simulink model "model_plane_identification_script_v1"  (R2015b)
settings: Solver=FixedStepDiscrete  StartTime=0.0  StopTime=20  RelTol=1e-3
values from neighbouring files (symbols this model uses):
  Aa = Amp_list(ii)    [amplitude_influence.m]    (also in datas.m = 1; model_validation.m = Amp_aileron2)
  Ae = Amp_list(ii)    [amplitude_influence.m]    (also in datas.m = 1; model_validation.m = Amp_elevator2)
  Ar = Amp_list(ii)    [amplitude_influence.m]    (also in datas.m = 1; model_validation.m = Amp_rudder2)
  b = 59.74    [datas.m]
  cbar = 8.32    [datas.m]
  K_wind = [0 0 0 0 0 0]'    [datas.m]
  m = 288772    [datas.m]
  Offset_Accelerometer = 57*10^-6    (= 5.7e-05)    [datas.m]
  Offset_gyro = 0.15/180*pi    (= 0.00261799387799)    [datas.m]
  Offset_velocity_angles = 0.1/180*pi    (= 0.00174532925199)    [datas.m]
  S = 510.95    [datas.m]
  Ta = 6    [datas.m]
  Te = 4    [datas.m]
  test_aileron = 1    [datas.m]    (also in model_validation.m = aileron2)
  test_elevator = 4    [datas.m]    (also in model_validation.m = elevator2)
  test_rudder = 1    [datas.m]    (also in model_validation.m = rudder2)
  Tr = 2    [datas.m]
undefined symbols (not defined in the file or in its folder): airlib, B747, DiscIntNeverNeededParam, DT, sigbuilder_block
undefined symbols (not defined in the file): Cd_0_true, Cd_alpha_true, Cd_deltae_true, Cd_q_true, Cdih_true, Cl_0_true, CL_0_true, CL_alpha_true, Cl_b_true, Cl_deltaa_true, CL_deltae_true, Cl_deltar_true, Cl_p_true, CL_q_true, Cl_r_true, CLih_true, Cm_0_true, Cm_alpha_true, Cm_deltae_true, Cm_ih_true, Cm_q_true, Cn_0_true, Cn_b_true, Cn_deltaa_true, Cn_deltar_true, Cn_p_true, Cn_r_true, Cy_0_true, Cy_b_true, Cy_deltaa_true, Cy_deltar_true, Cy_p_true, Cy_r_true, Ix, Iy, Iz, Jxy, Jxz, Jyz, V
libraries: simulink x4
(part 2 of 2)

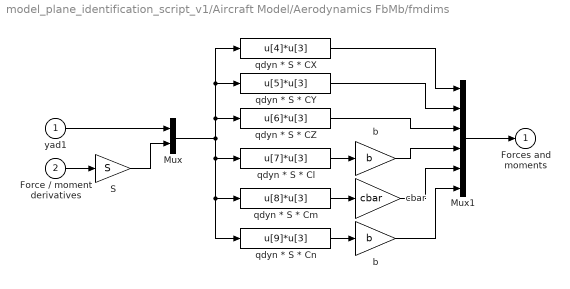
== system model_plane_identification_script_v1/Aircraft Model/Aerodynamics FbMb/fmdims ==
  yad1 : Inport
  Force / moment derivatives : Inport  Port=2
  Mux : Mux  Inputs=[3 6]
  Mux1 : Mux  Inputs=6
  S : Gain  Gain=S  SaturateOnIntegerOverflow=on  OutDataTypeStr=Inherit: Same as input  ParamDataTypeStr=Inherit: Same as input
  b : Gain  Gain=b  SaturateOnIntegerOverflow=on  OutDataTypeStr=Inherit: Same as input  ParamDataTypeStr=Inherit: Same as input
  "b " : Gain  Gain=b  SaturateOnIntegerOverflow=on  OutDataTypeStr=Inherit: Same as input  ParamDataTypeStr=Inherit: Same as input
  cbar : Gain  Gain=cbar  SaturateOnIntegerOverflow=on  OutDataTypeStr=Inherit: Same as input  ParamDataTypeStr=Inherit: Same as input
  qdyn * S * CX : Fcn  Expr=u[4]*u[3]
  qdyn * S * CY : Fcn  Expr=u[5]*u[3]
  qdyn * S * CZ : Fcn  Expr=u[6]*u[3]
  qdyn * S * Cl : Fcn  Expr=u[7]*u[3]
  qdyn * S * Cm : Fcn  Expr=u[8]*u[3]
  qdyn * S * Cn : Fcn  Expr=u[9]*u[3]
  Forces and moments : Outport
  wires:
  b/1 -> Mux1/4
  qdyn * S * CZ/1 -> Mux1/3
  S/1 -> Mux/2
  qdyn * S * CY/1 -> Mux1/2
  qdyn * S * CX/1 -> Mux1/1
  yad1/1 -> Mux/1
  qdyn * S * Cn/1 -> "b "/1
  qdyn * S * Cm/1 -> cbar/1
  qdyn * S * Cl/1 -> b/1
  Mux/1 -> qdyn * S * Cn/1, qdyn * S * Cm/1, qdyn * S * Cl/1, qdyn * S * CY/1, qdyn * S * CX/1, qdyn * S * CZ/1
  Force / moment derivatives/1 -> S/1
  cbar/1 -> Mux1/5
  "b "/1 -> Mux1/6
  Mux1/1 -> Forces and moments/1

== system model_plane_identification_script_v1/Aircraft Model/Aircraft equations of motion (General)/ODE ==
  x : Inport
  Ftot : Inport  Port=2
  Mtot : Inport  Port=3
  yhlp : Inport  Port=4
  ybvel* : Inport  Port=5
  Eulerdot : Subsystem  mask(Eulerdot){}
      mask help:
      | Calculation of d(psi)/dt, d(theta)/dt,
      | and d(phi/dt)
      mask Display: disp('psi dot\ntheta dot\nphi dot')
  Mux : Mux  Inputs=[12 3 3 11]
  Mux1 : Mux  Inputs=[3 3 3 3]
  Vabdot : Subsystem  mask(Vabdot){m=GM1(10)}
      mask prompts: m "Mass of the aircraft [kg]:"
      mask help: Calculation of dV/dt, dalpha/dt, dbeta/dt.
      mask Display: disp('V dot\nalpha dot\nbeta dot')
  pqrdot : Subsystem  mask(pqrdot){}
      mask help: Calculation of dp/dt, dq/dt, and dr/dt
      mask Display: disp('p dot\nq dot\nr dot')
  xyHdot : Subsystem  mask(xyHdot){}
      mask help: Calculation of d(xe)/dt, d(ye)/dt, and dH/dt
      mask Display: disp('xe dot\nye dot\nH dot')
  xdot : Outport
  wires:
  Mux1/1 -> xdot/1
  Vabdot/1(yVab) -> Mux1/1
  pqrdot/1(ypqr) -> Mux1/2
  Eulerdot/1(yeul) -> Mux1/3
  xyHdot/1(yxyH) -> Mux1/4
  yhlp/1 -> Mux/4
  ybvel*/1 -> xyHdot/1(ybvel*)
  Mux/1 -> xyHdot/2(uxYH), Eulerdot/1(ueul), Vabdot/1(uVab), pqrdot/1(upqr)
  Ftot/1 -> Mux/2
  Mtot/1 -> Mux/3
  x/1 -> Mux/1

== system model_plane_identification_script_v1/Aircraft Model/Aircraft equations of motion (General)/uvw ==
  yhlp : Inport
  x : Inport  Port=2
  Mux : Mux  Inputs=3
  Mux1 : Mux  Inputs=[12 11]
  u : Fcn  Expr=u[1]*u[13]*u[15]
  v : Fcn  Expr=u[1]*u[16]
  w : Fcn  Expr=u[1]*u[14]*u[15]
  ybvel : Outport
  wires:
  Mux/1 -> ybvel/1
  w/1 -> Mux/3
  v/1 -> Mux/2
  u/1 -> Mux/1
  x/1 -> Mux1/1
  yhlp/1 -> Mux1/2
  Mux1/1 -> v/1, w/1, u/1

== system model_plane_identification_script_v1/Aircraft Model/Aircraft equations of motion (General)/xdotcorr ==
  xdot uncorrected : Inport
  yhlp : Inport  Port=2
  yatm : Inport  Port=3
  Demux : Demux  Outputs=12
  Mux1 : Mux  Inputs=12
  Mux2 : Mux  Inputs=[11 1 5]
  beta dot correction : Fcn  Expr=u[12] / (1 - (u[3]*u[13]*b*S*CYbdot)/(4*m))
  xdot corrected : Outport
  wires:
  yhlp/1 -> Mux2/1
  Mux2/1 -> beta dot correction/1
  Mux1/1 -> xdot corrected/1
  xdot uncorrected/1 -> Demux/1
  Demux/3 -> Mux2/2
  Demux/12 -> Mux1/12
  Demux/11 -> Mux1/11
  Demux/10 -> Mux1/10
  Demux/9 -> Mux1/9
  Demux/8 -> Mux1/8
  Demux/7 -> Mux1/7
  Demux/6 -> Mux1/6
  Demux/5 -> Mux1/5
  Demux/4 -> Mux1/4
  Demux/2 -> Mux1/2
  Demux/1 -> Mux1/1
  yatm/1 -> Mux2/3
  beta dot correction/1 -> Mux1/3

== system model_plane_identification_script_v1/Aircraft Model/Airdata calculation/ad1 ==
  x : Inport
  yatm : Inport  Port=2
  Mach : Fcn  Expr=u[2]/u[1]
  Mux : Mux  Inputs=[1 12]
  Mux1 : Mux  Inputs=[12 5]
  Mux2 : Mux  Inputs=3
  dynamic pressure : Fcn  Expr=0.5*u[13]*u[1]^2
  soundspeed : Fcn  Expr=sqrt(401.8743*u[3])
  yad1 : Outport
  wires:
  yatm/1 -> Mux1/2, soundspeed/1
  x/1 -> Mux1/1, Mux/2
  Mux/1 -> Mach/1
  Mux1/1 -> dynamic pressure/1
  Mach/1 -> Mux2/2
  soundspeed/1 -> Mux2/1, Mux/1
  dynamic pressure/1 -> Mux2/3
  Mux2/1 -> yad1/1

== system model_plane_identification_script_v1/Aircraft Model/Airdata calculation/ad2 ==
  yatm : Inport
  yad1 : Inport  Port=2
  Mux : Mux  Inputs=[5 3]
  Mux1 : Mux  Inputs=3
  Vc : Fcn  Expr=sqrt(579000*((1+u[1]/101325)^(1/3.5)-1))
  Ve : Fcn  Expr=sqrt(u[8] * 1.63265)
  qc : Fcn  Expr=u[2] * ((1+0.2*u[7]^2)^3.5-1)
  yad2 : Outport
  wires:
  Mux1/1 -> yad2/1
  qc/1 -> Mux1/1, Vc/1
  Vc/1 -> Mux1/3
  Ve/1 -> Mux1/2
  Mux/1 -> Ve/1, qc/1
  yatm/1 -> Mux/1
  yad1/1 -> Mux/2

== system model_plane_identification_script_v1/Aircraft Model/Airdata calculation/ad3 ==
  x : Inport
  yatm : Inport  Port=2
  yad1 : Inport  Port=3
  Mux : Mux  Inputs=3
  Mux1 : Mux  Inputs=[12 5 3]
  Re : Fcn  Expr=(u[13]*u[1])/u[16]
  Tt : Fcn  Expr=u[15] * (1+0.2*u[19]^2)
  cbar : Gain  Gain=cbar  SaturateOnIntegerOverflow=on  OutDataTypeStr=Inherit: Same as input  ParamDataTypeStr=Inherit: Same as input
  yad3 : Outport
  wires:
  cbar/1 -> Mux/3
  Tt/1 -> Mux/1
  Mux/1 -> yad3/1
  Mux1/1 -> Tt/1, Re/1
  Re/1 -> cbar/1, Mux/2
  x/1 -> Mux1/1
  yatm/1 -> Mux1/2
  yad1/1 -> Mux1/3

== system model_plane_identification_script_v1/Aircraft Model/Airdata calculation/atm ==
  x : Inport
  Mux : Mux  Inputs=2
  Mux1 : Mux  Inputs=[2 1]
  Mux2 : Mux  Inputs=5
  T : Fcn  Expr=288.15 - 0.0065*u[12]
  g : Fcn  Expr=9.80665*(6371020/(6371020+u[12]))^2
  mu : Fcn  Expr=(1.458*10^(-6)*u[2]^1.5)/(u[2]+110.4)
  ps : Fcn  Expr=101325*(u[2]/288.15)^(u[1]/1.86584)
  rho : Fcn  Expr=u[3]/(287.053*u[2])
  yatm : Outport
  wires:
  mu/1 -> Mux2/4
  Mux2/1 -> yatm/1
  Mux1/1 -> rho/1
  rho/1 -> Mux2/1
  g/1 -> Mux2/5, Mux/1
  T/1 -> Mux2/3, Mux/2
  ps/1 -> Mux2/2, Mux1/2
  Mux/1 -> ps/1, mu/1, Mux1/1
  x/1 -> g/1, T/1

== system model_plane_identification_script_v1/Aircraft Model/Aerodynamics FbMb/aero/AM  ==
  In1 : Inport
  Matrix Gain : StateSpace  A=[]  B=[]  C=[]  D=M  X0=0
  Out1 : Outport
  wires:
  Matrix Gain/1 -> Out1/1
  In1/1 -> Matrix Gain/1

== system model_plane_identification_script_v1/Aircraft Model/Aerodynamics FbMb/aero/Stability 2 Body Axis ==
  alpha : Inport
  FsMb : Inport  Port=2
  Demux2 : Demux  Outputs=6
  Mux1 : Mux  Inputs=6
  Product{2..5} (4 alike) : Product  SaturateOnIntegerOverflow=on  RndMeth=Zero  InputSameDT=on  OutDataTypeStr=Inherit: Same as first input
  Sum3 : Sum  Inputs=-+  SaturateOnIntegerOverflow=on  InputSameDT=on  OutDataTypeStr=Inherit: Same as first input
  Sum4 : Sum  Inputs=--  SaturateOnIntegerOverflow=on  InputSameDT=on  OutDataTypeStr=Inherit: Same as first input
  cos alpha : Fcn  Expr=cos(u[1])
  sin alpha : Fcn
  FbMb : Outport
  wires:
  FsMb/1 -> Demux2/1
  Mux1/1 -> FbMb/1
  alpha/1 -> cos alpha/1, sin alpha/1
  Sum4/1 -> Mux1/3
  Product5/1 -> Sum4/2
  Product4/1 -> Sum4/1
  Demux2/3 -> Product5/2, Product3/2
  sin alpha/1 -> Product4/1, Product3/1
  Sum3/1 -> Mux1/1
  Product3/1 -> Sum3/2
  Product2/1 -> Sum3/1
  Demux2/1 -> Product4/2, Product2/2
  cos alpha/1 -> Product5/1, Product2/1
  Demux2/4 -> Mux1/4
  Demux2/2 -> Mux1/2
  Demux2/5 -> Mux1/5
  Demux2/6 -> Mux1/6

== system model_plane_identification_script_v1/Aircraft Model/Aircraft equations of motion (General)/ODE/Eulerdot ==
  note: yeul=[psi dot; theta dot; phi dot]
  note: ueul=[x;Ftot;Mtot;yhlp]
  ueul : Inport
  Mux1 : Mux  Inputs=[29 1]
  Mux2 : Mux  Inputs=3
  phi dot : Fcn  Expr=u[4] + u[30]*u[26]
  psi dot : Fcn  Expr=(u[5]*u[28] + u[6]*u[29])/u[27]
  theta dot : Fcn  Expr=u[5]*u[29] - u[6]*u[28]
  yeul : Outport
  wires:
  Mux1/1 -> phi dot/1
  phi dot/1 -> Mux2/3
  Mux2/1 -> yeul/1
  theta dot/1 -> Mux2/2
  psi dot/1 -> Mux1/2, Mux2/1
  ueul/1 -> psi dot/1, Mux1/1, theta dot/1

== system model_plane_identification_script_v1/Aircraft Model/Aircraft equations of motion (General)/ODE/Vabdot ==
  note: uVab=[x;Ftot;Mtot;yhlp]
  note: yVab=[V dot;alpha dot;beta dot]
  uVab : Inport
  Mux2 : Mux  Inputs=3
  V dot : Fcn  Expr=(u[13]*u[19]*u[21]+u[14]*u[22]+u[15]*u[20]*u[21])/m
  alpha dot : Fcn  Expr=(-u[13]*u[20]+u[15]*u[19])/(m*u[1]*u[21]) - u[23]*(u[4]*u[19]+u[6]*u[20]) + u[5]
  beta dot : Fcn  Expr=(-u[13]*u[19]*u[22]+u[14]*u[21]-u[15]*u[20]*u[22])/(m*u[1]) + u[4]*u[20] - u[6]*u[19]
  yVab : Outport
  wires:
  Mux2/1 -> yVab/1
  uVab/1 -> V dot/1, beta dot/1, alpha dot/1
  alpha dot/1 -> Mux2/2
  V dot/1 -> Mux2/1
  beta dot/1 -> Mux2/3

== system model_plane_identification_script_v1/Aircraft Model/Aircraft equations of motion (General)/ODE/pqrdot ==
  note: [p q r]'
  note: [L M N]'
  note: Here: ypqr = GM2*ytmp
  note: ytmp
  note: ypqr=[p dot;q dot;r dot]
  note: upqr=[x;Ftot;Mtot;yhlp]
  note: ytmp = [L; M; N; p^2; pq; pr; q^2; qr; r^2]
  upqr : Inport
  Demux : Demux  Outputs=[3 3 9 3 11]
  Fcn : Fcn  Expr=u[1]^2
  Fcn1 : Fcn  Expr=u[1]*u[2]
  Fcn2 : Fcn  Expr=u[1]*u[3]
  Fcn3 : Fcn  Expr=u[2]^2
  Fcn4 : Fcn  Expr=u[2]*u[3]
  Fcn5 : Fcn  Expr=u[3]^2
  "GM2 " : Subsystem  mask(State Space){M=GM2}
      mask prompts: M "Matrix"
      mask Display: disp('Matrix\nGain')
  Mux : Mux  Inputs=[3 1 1 1 1 1 1]
  Terminator1 : Terminator
  Terminator2 : Terminator
  Terminator3 : Terminator
  ypqr : Outport
  wires:
  upqr/1 -> Demux/1
  Demux/1 -> Terminator3/1
  Demux/5 -> Terminator2/1
  Demux/3 -> Terminator1/1
  Demux/2 -> Fcn1/1, Fcn/1, Fcn2/1, Fcn4/1, Fcn5/1, Fcn3/1
  Demux/4 -> Mux/1
  Fcn/1 -> Mux/2
  Fcn1/1 -> Mux/3
  Fcn2/1 -> Mux/4
  Fcn3/1 -> Mux/5
  Fcn4/1 -> Mux/6
  Fcn5/1 -> Mux/7
  "GM2 "/1(Out1) -> ypqr/1
  Mux/1 -> "GM2 "/1(In1)

== system model_plane_identification_script_v1/Aircraft Model/Aircraft equations of motion (General)/ODE/xyHdot ==
  note: yxyH=[xe dot; ye dot; H dot]
  note: uxyH=[x;Ftot;Mtot;yhlp]
  ybvel* : Inport
  uxYH : Inport  Port=2
  H dot : Fcn  Expr=u[30]*u[26] - (u[31]*u[28]+u[32]*u[29])*u[27]
  Mux2 : Mux  Inputs=[29 3]
  Mux3 : Mux  Inputs=2
  Mux4 : Mux  Inputs=[29 2]
  Mux5 : Mux  Inputs=3
  tmp1 : Fcn  Expr=u[30]*u[27] + (u[31]*u[28]+u[32]*u[29])*u[26]
  tmp2 : Fcn  Expr=u[31]*u[29] - u[32]*u[28]
  xe dot : Fcn  Expr=u[30]*u[25] - u[31]*u[24]
  ye dot : Fcn  Expr=u[30]*u[24] + u[31]*u[25]
  yxyH : Outport
  wires:
  tmp1/1 -> Mux3/1
  H dot/1 -> Mux5/3
  xe dot/1 -> Mux5/1
  tmp2/1 -> Mux3/2
  ye dot/1 -> Mux5/2
  Mux5/1 -> yxyH/1
  Mux4/1 -> ye dot/1, xe dot/1
  Mux2/1 -> H dot/1, tmp2/1, tmp1/1
  Mux3/1 -> Mux4/2
  ybvel*/1 -> Mux2/2
  uxYH/1 -> Mux4/1, Mux2/1

== system model_plane_identification_script_v1/Aircraft Model/Aircraft equations of motion (General)/ODE/pqrdot/GM2  ==
  In1 : Inport
  Matrix Gain : StateSpace  A=[]  B=[]  C=[]  D=M  X0=0
  Out1 : Outport
  wires:
  Matrix Gain/1 -> Out1/1
  In1/1 -> Matrix Gain/1

== matlab function model_plane_identification_script_v1/CL/pilot__aileron_command/input1 ==
  data: u input; y output; T input; A input
function y = input211(u,T,A)

if ((u>=T) && (u<(T+1)))
    y= A ;
elseif ((u>=(T+1)) && (u<(T+1.5)))
    y=-A; 
elseif ((u>=(T+1.5)) && (u<(T+2)))
    y=A;    
else
    y=0;
end

== matlab function model_plane_identification_script_v1/CL/pilot__aileron_command/input11 ==
  data: u input; y output; T input; A input
function y = input11(u,T,A)
if ((u>=T) && (u<(T+1)))
    y=A;
elseif ((u>=(T+1)) && (u<(T+2)))
    y=-A;   
else
    y=0;
end

== matlab function model_plane_identification_script_v1/CL/pilot__aileron_command/input3211 ==
  data: u input; y output; T input; A input
function y = input3211(u,T,A)
if ((u>=T) && (u<(T+1)))
    y=A;
elseif ((u>=(T+1)) && (u<(T+1.5)))
    y=-A; 
elseif ((u>=(T+1.5)) && (u<(T+1.75)))
    y=A;   
elseif ((u>=(T+1.75)) && (u<(T+2)))
    y=-A;   
else
    y=0;
end

== matlab function model_plane_identification_script_v1/CL/pilot_rudder_command/input1 ==
  data: u input; y output; T input; A input
function y = input211(u,T,A)

if ((u>=T) && (u<(T+1)))
    y=A;
elseif ((u>=(T+1)) && (u<(T+1.5)))
    y=-A; 
elseif ((u>=(T+1.5)) && (u<(T+2)))
    y=A;    
else
    y=0;
end

== matlab function model_plane_identification_script_v1/CL/pilot_rudder_command/input11 ==
  data: u input; y output; T input; A input
function y = input11(u,T,A)
if ((u>=T) && (u<(T+1)))
    y=A;
elseif ((u>=(T+1)) && (u<(T+2)))
    y=-A;   
else
    y=0;
end

== matlab function model_plane_identification_script_v1/CL/pilot_rudder_command/input3211 ==
  data: u input; y output; T input; A input
function y = input3211(u,T,A)
if ((u>=T) && (u<(T+1)))
    y=A;
elseif ((u>=(T+1)) && (u<(T+1.5)))
    y=-A; 
elseif ((u>=(T+1.5)) && (u<(T+1.75)))
    y=A;   
elseif ((u>=(T+1.75)) && (u<(T+2)))
    y=-A;   
else
    y=0;
end

== matlab function model_plane_identification_script_v1/CL/pilot__elevator_command/input211 ==
  data: u input; y output; T input; A input
function y = input211(u,T,A)

if ((u>=T) && (u<(T+1)))
    y=A;
elseif ((u>=(T+1)) && (u<(T+1.5)))
    y=-A; 
elseif ((u>=(T+1.5)) && (u<(T+2)))
    y=A;    
else
    y=0;
end

== matlab function model_plane_identification_script_v1/CL/pilot__elevator_command/input11 ==
  data: u input; y output; T input; A input
function y = input11(u,T,A)
if ((u>=T) && (u<(T+1)))
    y=A;
elseif ((u>=(T+1)) && (u<(T+2)))
    y=-A;   
else
    y=0;
end

== matlab function model_plane_identification_script_v1/CL/pilot__elevator_command/input3211 ==
  data: u input; y output; T input; A input
function y = input3211(u,T,A)

if ((u>=T) && (u<(T+1)))
    y=A;
elseif ((u>=(T+1)) && (u<(T+1.5)))
    y=-A; 
elseif ((u>=(T+1.5)) && (u<(T+1.75)))
    y=A;    
elseif ((u>=(T+1.75)) && (u<(T+2)))
    y=-A;  
else
    y=0;
end
